simulink model "beam_control_ic_rx"  (R2022b)
settings: Solver=VariableStepAuto  StartTime=0.0  StopTime=136e-9  RelTol=1e-3
values from neighbouring files (symbols this model uses):
  Bias = 0    [ModelingRFSystemsWithAntennaArraysUsingAntennaBlockExample.m]    (also in beam_control_ic_rx_parameter.m)
  filter_gain0_0 = 0    [ModelingRFSystemsWithAntennaArraysUsingAntennaBlockExample.m]    (also in beam_control_ic_rx_parameter.m)
  filter_gain0_1 = 1/6    (= 0.166666666667)    [ModelingRFSystemsWithAntennaArraysUsingAntennaBlockExample.m]    (also in beam_control_ic_rx_parameter.m)
  filter_gain0_2 = 2/3    (= 0.666666666667)    [ModelingRFSystemsWithAntennaArraysUsingAntennaBlockExample.m]    (also in beam_control_ic_rx_parameter.m)
  filter_gain0_3 = 1/6    (= 0.166666666667)    [ModelingRFSystemsWithAntennaArraysUsingAntennaBlockExample.m]    (also in beam_control_ic_rx_parameter.m)
  filter_gain1_0 = 0    [ModelingRFSystemsWithAntennaArraysUsingAntennaBlockExample.m]    (also in beam_control_ic_rx_parameter.m)
  filter_gain1_1 = 1/2    (= 0.5)    [ModelingRFSystemsWithAntennaArraysUsingAntennaBlockExample.m]    (also in beam_control_ic_rx_parameter.m)
  filter_gain1_2 = 0    [ModelingRFSystemsWithAntennaArraysUsingAntennaBlockExample.m]    (also in beam_control_ic_rx_parameter.m)
  filter_gain1_3 = -1/2    (= -0.5)    [ModelingRFSystemsWithAntennaArraysUsingAntennaBlockExample.m]    (also in beam_control_ic_rx_parameter.m)
  filter_gain2_0 = 0    [ModelingRFSystemsWithAntennaArraysUsingAntennaBlockExample.m]    (also in beam_control_ic_rx_parameter.m)
  filter_gain2_1 = 1/2    (= 0.5)    [ModelingRFSystemsWithAntennaArraysUsingAntennaBlockExample.m]    (also in beam_control_ic_rx_parameter.m)
  filter_gain2_2 = -1    [ModelingRFSystemsWithAntennaArraysUsingAntennaBlockExample.m]    (also in beam_control_ic_rx_parameter.m)
  filter_gain2_3 = 1/2    (= 0.5)    [ModelingRFSystemsWithAntennaArraysUsingAntennaBlockExample.m]    (also in beam_control_ic_rx_parameter.m)
  filter_gain3_0 = 1/6    (= 0.166666666667)    [ModelingRFSystemsWithAntennaArraysUsingAntennaBlockExample.m]    (also in beam_control_ic_rx_parameter.m)
  filter_gain3_1 = -1/2    (= -0.5)    [ModelingRFSystemsWithAntennaArraysUsingAntennaBlockExample.m]    (also in beam_control_ic_rx_parameter.m)
  filter_gain3_2 = 1/2    (= 0.5)    [ModelingRFSystemsWithAntennaArraysUsingAntennaBlockExample.m]    (also in beam_control_ic_rx_parameter.m)
  filter_gain3_3 = -1/6    (= -0.166666666667)    [ModelingRFSystemsWithAntennaArraysUsingAntennaBlockExample.m]    (also in beam_control_ic_rx_parameter.m)
  fraction_delay = 1.5    [ModelingRFSystemsWithAntennaArraysUsingAntennaBlockExample.m]    (also in beam_control_ic_rx_parameter.m = 1)
  integer_delay = 0    [ModelingRFSystemsWithAntennaArraysUsingAntennaBlockExample.m]    (also in beam_control_ic_rx_parameter.m)
  N = 10    [ModelingRFSystemsWithAntennaArraysUsingAntennaBlockExample.m]    (also in beam_control_ic_rx_parameter.m)
  Ref = 2.048    [ModelingRFSystemsWithAntennaArraysUsingAntennaBlockExample.m]    (also in beam_control_ic_rx_parameter.m)
  rx_amplitude_compensation = 1    [ModelingRFSystemsWithAntennaArraysUsingAntennaBlockExample.m]    (also in beam_control_ic_rx_parameter.m)
  rx_freq_d_compensation = 250e6    (= 250000000)    [ModelingRFSystemsWithAntennaArraysUsingAntennaBlockExample.m]    (also in beam_control_ic_rx_parameter.m)
  rx_phase_compensation = 0    [ModelingRFSystemsWithAntennaArraysUsingAntennaBlockExample.m]    (also in beam_control_ic_rx_parameter.m)
undefined symbols (not defined in the file or in its folder): fdesignblkfcn, gcbh, pskmod
libraries: dspsigops x5, simulink_extras x3, dspmlti4 x3, msbDacArchitectures x2, commrfcorlib x1, commeq3 x1
(part 1 of 3)
settings Model: Creator=BOBO  LastModifiedBy=BOBO

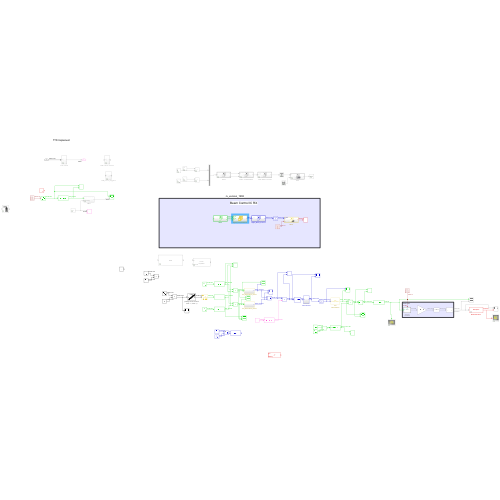
[thumbnail: Simulink's stored preview of the top-level diagram]
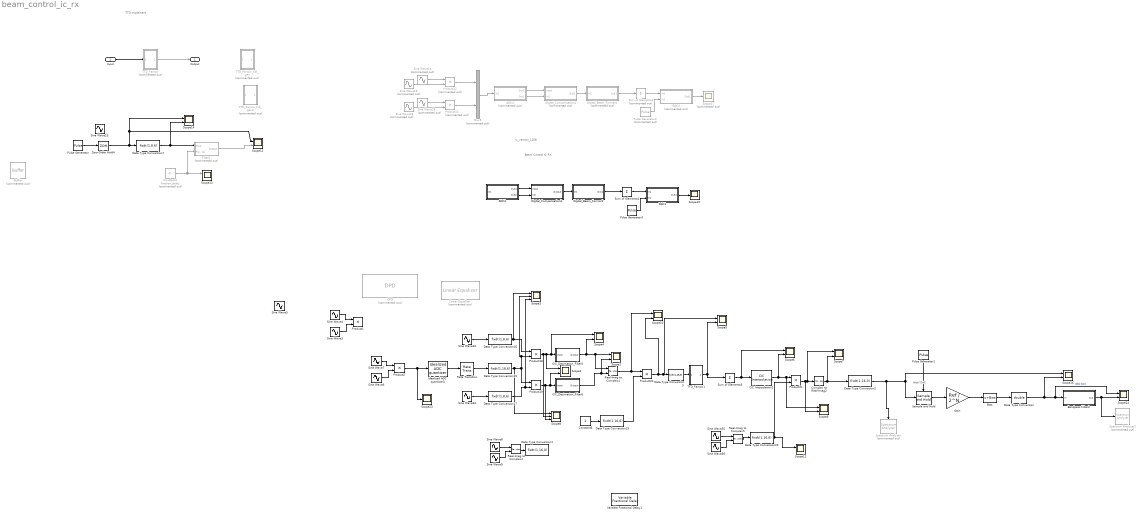
== system beam_control_ic_rx ==
  note: TTD Implement
  note: Ideal DAC
  note: rx_version_1208
  note: Beam Control IC RX
  Input : Inport
  ADC3 : Subsystem  TreatAsAtomicUnit=on
  ADC4 : Subsystem  Commented=on  TreatAsAtomicUnit=on
  Bandpass Filter3 : Subsystem  DialogController=fdesignblkfcn  InitFcn=fdesignblkfcn(gcbh, {'InitFcn'});  mask(Bandpass Filter){}
      mask help: Design a bandpass filter
      settings: CopyFcn=fdesignblkfcn(gcbh, {'CopyFcn'});
      mask Help: helpview(mapfilelocation('dsp'), 'dspbandpassfilter');
      mask Display: disp('Bandpass');
  Bias : Bias  Bias=Bias  SaturateOnIntegerOverflow=off
  Buffer : Buffer  Commented=on  OutputFrames=off
  CIC Interpolation2 : dspmlti4/CIC Interpolation  filtFrom=Dialog parameters  filtobj=Hm_interp  ftype=Interpolator  R=2  M=1  N=2  filterInternals=Full precision  BPS=[16 16 16 16]  FLPS=0  outputWordLength=32  outputFracLength=0  launchFVT=off  framing=Allow multirate processing  OutputFrames=off
      settings: LibrarySourceBlock=|
      | dsphdlsupportfiltering/CIC
      | Interpolation
  CIC_Decimation_Filter5 : Subsystem  Tag=FilterWizardSubSystem
      settings: ErrorFcn=dspFilterRealizedInBasicElemsAlgLoopErrFcnCallback
  CIC_Decimation_Filter6 : Subsystem  Tag=FilterWizardSubSystem
      settings: ErrorFcn=dspFilterRealizedInBasicElemsAlgLoopErrFcnCallback
  Complex to Real-Imag2 : ComplexToRealImag  Output=Real
  Constant4 : Constant  Commented=on  Value=fraction_delay  OutMin=0  OutMax=1  OutDataTypeStr=fixdt(1,16,10)
  Constant6 : Constant
  DAC3 : Subsystem  TreatAsAtomicUnit=on
  DAC4 : Subsystem  Commented=on  TreatAsAtomicUnit=on
  DPD : commrfcorlib/DPD  Commented=on  PolynomialType=Memory polynomial  CoefficientSource=Property  Coefficients=complex([1 0 0 0 0; 0 0 0 0 0; 0 0 0 0 0])  SimulateUsing=Code generation
  Data Type Conversion : DataTypeConversion  OutDataTypeStr=double  SaturateOnIntegerOverflow=off  RndMeth=Floor
  Data Type Conversion1 : DataTypeConversion  OutDataTypeStr=fixdt(1,16,0)  SaturateOnIntegerOverflow=off  RndMeth=Floor
  Data Type Conversion{3,15,19..20} (4 alike) : DataTypeConversion  OutDataTypeStr=fixdt(1,16,6)  SaturateOnIntegerOverflow=off  RndMeth=Floor
  Data Type Conversion16 : DataTypeConversion  OutDataTypeStr=fixdt(1,8,6)  SaturateOnIntegerOverflow=off  RndMeth=Floor
  Data Type Conversion17 : DataTypeConversion  OutDataTypeStr=fixdt(1,8,6)  SaturateOnIntegerOverflow=off  RndMeth=Floor
  Data Type Conversion2 : DataTypeConversion  OutDataTypeStr=fixdt(1,16,0)  SaturateOnIntegerOverflow=off  RndMeth=Floor
  Data Type Conversion7 : DataTypeConversion  OutMin=-1  OutMax=0.99  OutDataTypeStr=fixdt(1,8,6)  SaturateOnIntegerOverflow=off  RndMeth=Floor
  Digital_Beam_Former3 : Subsystem  TreatAsAtomicUnit=on
  Digital_Beam_Former4 : Subsystem  Commented=on  TreatAsAtomicUnit=on
  Digital_Compensation3 : Subsystem  TreatAsAtomicUnit=on
  Digital_Compensation4 : Subsystem  Commented=on  TreatAsAtomicUnit=on
  Filter1 : Subsystem  Tag=FilterWizardSubSystem  Commented=on
      settings: ErrorFcn=dspFilterRealizedInBasicElemsAlgLoopErrFcnCallback
  Gain : Gain  Gain=Ref / 2^N
  Idealized ADC quantizer3 : simulink_extras/Additional Discrete/Idealized ADC quantizer  NumberOfConverterBits=8  Vmin=-1  Vmax=1  OutputDataType=double  OutputNegativeValues=on
  Linear Equalizer : commeq3/Linear Equalizer  Commented=on  NumTaps=5  Constellation=pskmod( 0:3, 4, pi/4, 'bin' )  InputSamplesPerSymbol=1  Algorithm=LMS  StepSize=0.01  ForgettingFactor=0.99  InitialInverseCorrelationMatrix=0.1  ReferenceTap=3  InputDelay=0  AdaptWeightsSource=Property  AdaptWeights=on  InitialWeightsSource=Auto  InitialWeights=0  TrainingInitialWeights=0  BlindInitialWeights=[ 0; 0; 1; 0; 0 ]  WeightUpdatePeriod=1  TrainingFlagInputPort=off  AdaptAfterTraining=on  ResetInputPort=off  ErrorOutputPort=off  TapWeightsOutputPort=off  SimulateUsing=Code generation
  Mux5 : Mux  Commented=on  Inputs=2
  Product{1..2,18..21} (6 alike) : Product
  Product11 : Product  Commented=on
  Product12 : Product  Commented=on
  Pulse Generator : DiscretePulseGenerator  PulseType=Time based  Period=5e-9  PulseWidth=50
  Pulse Generator1 : DiscretePulseGenerator  PulseType=Time based  Period=1/1e9  PulseWidth=50
  Pulse Generator2 : DiscretePulseGenerator  Commented=on  PulseType=Time based  Period=1/1e9  PulseWidth=50
  Pulse Generator3 : DiscretePulseGenerator  PulseType=Time based  Period=1/1e9  PulseWidth=50
  Rate Transition : RateTransition  OutPortSampleTime=1/1e9
  Real-Imag to Complex2 : RealImagToComplex
  Real-Imag to Complex4 : RealImagToComplex
  Real-Imag to Complex5 : RealImagToComplex
  Sample and Hold : dspsigops/Sample and Hold  trig=Rising edge  initCond=0  latchinput=off
  Scope{1..2,4..7,9..14,16,24} (14 alike) : Scope  NumInputPorts=2
  Scope15 : Scope
  Scope17 : Scope  Commented=on
  Scope23 : Scope
  Scope3 : Scope  NumInputPorts=3
  Scope8 : Scope  NumInputPorts=3
  Sine Wave14 : Sin  Commented=on  Frequency=2*pi*3.25e9  SampleTime=0
  Sine Wave19 : Sin  Commented=on  Frequency=2*pi*62.5e6  SampleTime=0
  Sine Wave23 : Sin  Frequency=2*pi*3.25e9  SampleTime=1e-11
  Sine Wave24 : Sin  Commented=on  Frequency=2*pi*3.25e9  SampleTime=0
  Sine Wave26 : Sin  Commented=on  Frequency=2*pi*62.5e6  SampleTime=0
  Sine Wave3 : Sin  Frequency=2*pi*62.5e6  SampleTime=0
  Sine Wave33 : Sin  Frequency=2*pi*250e6  Phase=1.57  SampleTime=1/1e9
  Sine Wave34 : Sin  Frequency=2*pi*250e6  SampleTime=1/1e9
  Sine Wave35 : Sin  Frequency=2*pi*250e6  Phase=1.57  SampleTime=1/1e9
  Sine Wave36 : Sin  Frequency=2*pi*250e6  SampleTime=1/1e9
  Sine Wave4 : Sin  Frequency=2*pi*3.25e9  SampleTime=0
  Sine Wave5 : Sin  Frequency=2*pi*3.25e9  SampleTime=0
  Sine Wave6 : Sin  Frequency=2*pi*62.5e6  SampleTime=0
  Sine Wave7 : Sin  Frequency=2*pi*3.25e9  SampleTime=0
  Sine Wave8 : Sin  Amplitude=rx_amplitude_compensation  Frequency=2*pi*rx_freq_d_compensation  Phase=pi*(rx_phase_compensation+90)/180  SampleTime=1/5e8
  Sine Wave9 : Sin  Amplitude=rx_amplitude_compensation  Frequency=2*pi*rx_freq_d_compensation  Phase=pi*rx_phase_compensation/180  SampleTime=1/5e8
  Spectrum Analyzer : SpectrumAnalyzer  Commented=on
  Spectrum Analyzer2 : SpectrumAnalyzer  Commented=on
  Sum of Elements1 : Sum  Inputs=+
  Sum of Elements4 : Sum  Commented=on  Inputs=+
  Sum of Elements5 : Sum  Inputs=+
  TTD_Farrow : Subsystem  Commented=on
  TTD_Farrow1 : Subsystem
  TTD_Farrow_hdl_gen : Subsystem  Commented=on
  TTD_Farrow_hdl_gen2 : Subsystem  Commented=on
  Variable Fractional Delay1 : dspsigops/Variable Fractional Delay  mode=OBSOLETE  modeActive=Linear  L=4  FarrowL=4  R=10  alpha=1  dmax=100  InputProcessing=Columns as channels (frame based)  ic=0  noDFT=off  fallbackFIR=Clip to the minimum value necessary for centered kernel  fallbackFarrow=Clip to the minimum value necessary for centered kernel  roundingMode=Zero  overflowMode=off
  Zero-Order Hold4 : ZeroOrderHold  SampleTime=1e-9
  Output : Outport
  wires:
  Input/1 -> TTD_Farrow/1(In1)
  TTD_Farrow/1(Output) -> Output/1
  Pulse Generator/1 -> Zero-Order Hold4/1
  Data Type Conversion7/1 -> Filter1/1(Input), Scope14/2
  Filter1/1(Output) -> Scope12/2
  Zero-Order Hold4/1 -> Scope14/1, Scope12/1, Data Type Conversion7/1
  Constant4/1 -> Filter1/2(FracDelay), Scope13/1
  Idealized ADC quantizer3/1 -> Rate Transition/1
  Rate Transition/1 -> Data Type Conversion15/1
  Sine Wave33/1 -> Data Type Conversion16/1
  Sine Wave34/1 -> Data Type Conversion17/1
  Data Type Conversion16/1 -> Product18/1, Scope3/1
  Data Type Conversion15/1 -> Scope8/1, Product19/1, Product18/2, Scope3/2
  Data Type Conversion17/1 -> Scope3/3, Product19/2
  Product18/1 -> Scope2/1, Scope4/1, CIC_Decimation_Filter5/1(Input), Scope8/2
  Product19/1 -> Scope8/3, Scope2/2, CIC_Decimation_Filter6/1(Input)
  CIC_Decimation_Filter5/1(Output) -> Scope4/2, Real-Imag to Complex4/1, Scope1/1
  CIC_Decimation_Filter6/1(Output) -> Scope1/2, Real-Imag to Complex4/2
  Real-Imag to Complex4/1 -> Scope10/1, Product20/1
  Data Type Conversion19/1 -> Product20/2
  Constant6/1 -> Data Type Conversion19/1
  Product20/1 -> Scope10/2, Scope5/1, Data Type Conversion3/1
  Sum of Elements5/1 -> Scope6/1, CIC Interpolation2/1
  CIC Interpolation2/1 -> Scope6/2, Scope9/1, Product21/1
  Sine Wave35/1 -> Real-Imag to Complex5/1
  Real-Imag to Complex5/1 -> Data Type Conversion20/1
  Sine Wave36/1 -> Real-Imag to Complex5/2
  Product21/1 -> Scope9/2, Scope7/1, Complex to Real-Imag2/1
  Complex to Real-Imag2/1 -> Scope7/2, Data Type Conversion2/1
  Pulse Generator1/1 -> Sample and Hold/Trigger
  Gain/1 -> Bias/1
  Bias/1 -> Data Type Conversion/1
  Sample and Hold/1 -> Gain/1
  Data Type Conversion2/1 -> Scope16/1, Sample and Hold/1, Spectrum Analyzer/1
  Data Type Conversion/1 -> Scope16/2, Scope24/1, Bandpass Filter3/1(In)  "Ideal DAC"
  Product12/1 -> Mux5/1
  Sine Wave14/1 -> Product12/1
  Sine Wave19/1 -> Product12/2
  Sine Wave26/1 -> Product11/2
  Sine Wave24/1 -> Product11/1
  Product11/1 -> Mux5/2
  Mux5/1 -> ADC4/1(In1)
  Digital_Compensation4/1(Out1) -> Digital_Beam_Former4/1(In1)
  ADC4/2(Out2) -> Digital_Compensation4/2(In2)
  ADC4/1(Out1) -> Digital_Compensation4/1(Input)
  DAC4/1(Out1) -> Scope17/1
  Sum of Elements4/1 -> DAC4/1(In1)
  Digital_Beam_Former4/1(Out1) -> Sum of Elements4/1
  Bandpass Filter3/1(Out) -> Spectrum Analyzer2/1, Scope24/2
  Pulse Generator2/1 -> DAC4/2(In2)
  Sine Wave3/1 -> Product1/2
  Sine Wave4/1 -> Product1/1
  Digital_Beam_Former3/1(Out1) -> Sum of Elements1/1
  Pulse Generator3/1 -> DAC3/2(In2)
  DAC3/1(Out1) -> Scope15/1
  Digital_Compensation3/1(Output) -> Digital_Beam_Former3/1(In1)
  Sum of Elements1/1 -> DAC3/1(In1)
  ADC3/2(Out2) -> Digital_Compensation3/2(In2)
  ADC3/1(Out1) -> Digital_Compensation3/1(Input)
  Data Type Conversion20/1 -> Product21/2, Scope11/1
  Sine Wave7/1 -> Product2/1
  Sine Wave6/1 -> Product2/2
  Product2/1 -> Scope23/1, Idealized ADC quantizer3/1
  Sine Wave8/1 -> Real-Imag to Complex2/1
  Sine Wave9/1 -> Real-Imag to Complex2/2
  Real-Imag to Complex2/1 -> Data Type Conversion1/1
  Data Type Conversion3/1 -> TTD_Farrow1/1(In1)
  TTD_Farrow1/1(Output) -> Sum of Elements5/1, Scope5/2

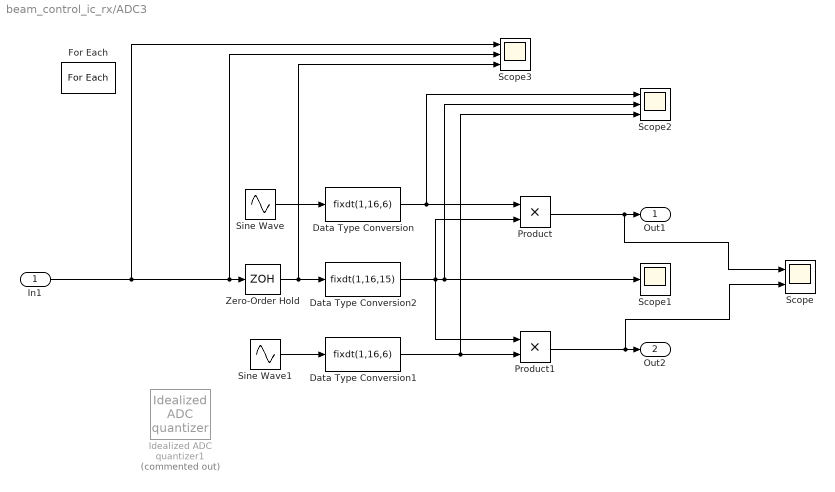
== system beam_control_ic_rx/ADC3 ==
  In1 : Inport  Partition=on  PartitionDimension=1  PartitionWidth=1  PartitionOffset=0
  Data Type Conversion : DataTypeConversion  OutMin=-1  OutMax=1  OutDataTypeStr=fixdt(1,16,6)  SaturateOnIntegerOverflow=off  RndMeth=Floor
  Data Type Conversion1 : DataTypeConversion  OutMin=-1  OutMax=1  OutDataTypeStr=fixdt(1,16,6)  SaturateOnIntegerOverflow=off  RndMeth=Floor
  Data Type Conversion2 : DataTypeConversion  OutMin=-1  OutMax=0.9  OutDataTypeStr=fixdt(1,16,15)  SaturateOnIntegerOverflow=off  RndMeth=Floor
  For Each : ForEach  DisableCoverage=on
  Idealized ADC quantizer1 : simulink_extras/Additional Discrete/Idealized ADC quantizer  Commented=on  NumberOfConverterBits=12  Vmin=-5  Vmax=5  OutputDataType=double  OutputNegativeValues=on
  Product : Product
  Product1 : Product
  Scope : Scope  NumInputPorts=2
  Scope1 : Scope
  Scope2 : Scope  NumInputPorts=3
  Scope3 : Scope  NumInputPorts=3
  Sine Wave : Sin  Frequency=2*pi*250e6  Phase=1.57  SampleTime=1/1e9
  Sine Wave1 : Sin  Frequency=2*pi*250e6  SampleTime=1/1e9
  Zero-Order Hold : ZeroOrderHold  SampleTime=1/1e9
  Out1 : Outport  ConcatenationDimension=1
  Out2 : Outport  Port=2  ConcatenationDimension=1
  wires:
  Data Type Conversion1/1 -> Scope2/3, Product1/2
  In1/1 -> Scope3/2, Zero-Order Hold/1, Scope3/1
  Sine Wave/1 -> Data Type Conversion/1
  Sine Wave1/1 -> Data Type Conversion1/1
  Zero-Order Hold/1 -> Scope3/3, Data Type Conversion2/1
  Data Type Conversion/1 -> Product/1, Scope2/1
  Data Type Conversion2/1 -> Scope1/1, Scope2/2, Product1/1, Product/2
  Product/1 -> Scope/1, Out1/1
  Product1/1 -> Scope/2, Out2/1

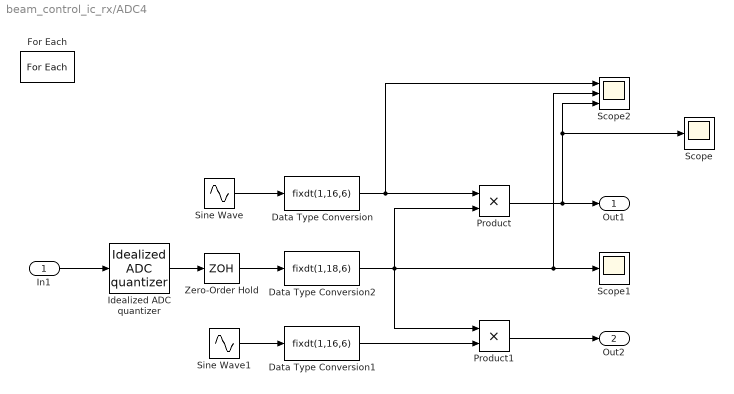
== system beam_control_ic_rx/ADC4 ==
  In1 : Inport  Partition=on  PartitionDimension=1  PartitionWidth=1  PartitionOffset=0
  Data Type Conversion : DataTypeConversion  OutMin=-1  OutMax=1  OutDataTypeStr=fixdt(1,16,6)  SaturateOnIntegerOverflow=off  RndMeth=Floor
  Data Type Conversion1 : DataTypeConversion  OutMin=-1  OutMax=1  OutDataTypeStr=fixdt(1,16,6)  SaturateOnIntegerOverflow=off  RndMeth=Floor
  Data Type Conversion2 : DataTypeConversion  OutMin=-2048  OutMax=2047  OutDataTypeStr=fixdt(1,18,6)  SaturateOnIntegerOverflow=off  RndMeth=Floor
  For Each : ForEach  DisableCoverage=on
  Idealized ADC quantizer : simulink_extras/Additional Discrete/Idealized ADC quantizer  NumberOfConverterBits=12  Vmin=-1  Vmax=1  OutputDataType=double  OutputNegativeValues=on
  Product : Product
  Product1 : Product
  Scope : Scope
  Scope1 : Scope
  Scope2 : Scope  NumInputPorts=3
  Sine Wave : Sin  Frequency=2*pi*250e6  Phase=1.57  SampleTime=1/1e9
  Sine Wave1 : Sin  Frequency=2*pi*250e6  SampleTime=1/1e9
  Zero-Order Hold : ZeroOrderHold  SampleTime=1/1e9
  Out1 : Outport  ConcatenationDimension=1
  Out2 : Outport  Port=2  ConcatenationDimension=1
  wires:
  Product1/1 -> Out2/1
  Product/1 -> Scope/1, Scope2/3, Out1/1
  Data Type Conversion2/1 -> Product/2, Product1/1, Scope2/2, Scope1/1
  Data Type Conversion/1 -> Scope2/1, Product/1
  Zero-Order Hold/1 -> Data Type Conversion2/1
  Sine Wave1/1 -> Data Type Conversion1/1
  Sine Wave/1 -> Data Type Conversion/1
  Idealized ADC quantizer/1 -> Zero-Order Hold/1
  In1/1 -> Idealized ADC quantizer/1
  Data Type Conversion1/1 -> Product1/2

== system beam_control_ic_rx/Bandpass Filter3 ==
  In : Inport
  Generated Filter Block : DiscreteFir  Tag=BlockMethodSubSystem  Coefficients=[-0.000551445390270867506 0.000407430436883946413 0.00151170095910276784 0.00170809108636746755 -0.000183233989486140172 -0.00314427517439309695 -0.00408384949539862194 -0.000859536641631024833 0.00458828280495307203 0.00703118910578414639 0.00304274168675388234 -0.00462111674625677576 -0.00882607470501511893 -0.00522014043057489156 0.00277191525149639382 0.00730259808984131537 0.00474853789832731764 -0.000332137279825720844 -0.00125943108082663064 0.001596135152078317 0.000647809790796010439 -0.00801520700503077603 -0.0156681967330769729 -0.00792830354994228381 0.0163284487042885569 0.0360058824865698776 0.0248375883164067765 -0.0180029551213413963 -0.0572925026311378038 -0.0501414407980040541 0.00875479098791274307 0.0720308491137559154 0.0780256286801277177 0.0114831560658058014 -0.0739106277220435842 -0.0999313296142419205 -0.0376048498748084298 0.0611143159293767238 0.108245533083798362 0.0611143159293767238 -0.0376048498748084298 -0.0999313296142419205 -0.0739106277220435842 0.0114831560658058014 0.0780256286801277177 0.0720308491137559154 0.00875479098791274307 -0.0501414407980040541 -0.0572925026311378038 -0.0180029551213413963 0.0248375883164067765 0.0360058824865698776 0.0163284487042885569 -0.00792830354994228381 -0.0156681967330769729 -0.00801520700503077603 0.000647809790796010439 0.001596135152078317 -0.00125943108082663064 -0.000332137279825720844 0.00474853789832731764 0.00730259808984131537 0.00277191525149639382 -0.00522014043057489156 -0.00882607470501511893 -0.00462111674625677576 0.00304274168675388234 0.00703118910578414639 0.00458828280495307203 -0.000859536641631024833 -0.00408384949539862194 -0.00314427517439309695 -0.000183233989486140172 0.00170809108636746755 0.00151170095910276784 0.000407430436883946413 -0.000551445390270867506]  InputProcessing=Columns as channels (frame based)
  Out : Outport  VectorParamsAs1DForOutWhenUnconnected=off
  wires:
  Generated Filter Block/1 -> Out/1
  In/1 -> Generated Filter Block/1

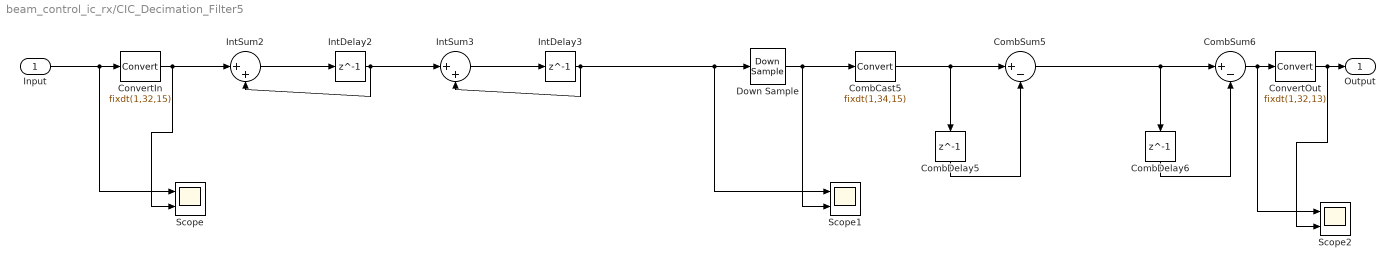
== system beam_control_ic_rx/CIC_Decimation_Filter5 ==
  Input : Inport
  CombCast5 : DataTypeConversion  OutDataTypeStr=fixdt(1,34,15)  SaturateOnIntegerOverflow=off  RndMeth=Floor
  CombDelay5 : Delay  DelayLength=1  InitialCondition=0
  CombDelay6 : Delay  DelayLength=1  InitialCondition=0
  CombSum5 : Sum  Inputs=|+-  AccumDataTypeStr=fixdt(1,34,15)  OutDataTypeStr=fixdt(1,34,15)
  CombSum6 : Sum  Inputs=|+-  AccumDataTypeStr=fixdt(1,34,15)  OutDataTypeStr=fixdt(1,34,15)
  ConvertIn : DataTypeConversion  OutDataTypeStr=fixdt(1,32,15)  RndMeth=Nearest
  ConvertOut : DataTypeConversion  OutDataTypeStr=fixdt(1,32,13)  SaturateOnIntegerOverflow=off  RndMeth=Floor
  Down Sample : DownSample  RateOptions=Allow multirate processing  AllowArbitraryFixedInput=on
  IntDelay2 : Delay  DelayLength=1  InitialCondition=0
  IntDelay3 : Delay  DelayLength=1  InitialCondition=0
  IntSum2 : Sum  Inputs=|++  AccumDataTypeStr=fixdt(1,34,15)  OutDataTypeStr=fixdt(1,34,15)
  IntSum3 : Sum  Inputs=|++  AccumDataTypeStr=fixdt(1,34,15)  OutDataTypeStr=fixdt(1,34,15)
  Scope : Scope  NumInputPorts=2
  Scope1 : Scope  NumInputPorts=2
  Scope2 : Scope  NumInputPorts=2
  Output : Outport
  wires:
  Input/1 -> Scope/1, ConvertIn/1
  ConvertIn/1 -> Scope/2, IntSum2/1
  IntSum2/1 -> IntDelay2/1
  IntDelay2/1 -> IntSum2/2, IntSum3/1
  IntSum3/1 -> IntDelay3/1
  IntDelay3/1 -> IntSum3/2, Scope1/1, Down Sample/1
  Down Sample/1 -> Scope1/2, CombCast5/1
  CombSum5/1 -> CombSum6/1, CombDelay6/1
  CombDelay5/1 -> CombSum5/2
  CombCast5/1 -> CombSum5/1, CombDelay5/1
  CombSum6/1 -> Scope2/1, ConvertOut/1
  CombDelay6/1 -> CombSum6/2
  ConvertOut/1 -> Scope2/2, Output/1

== system beam_control_ic_rx/CIC_Decimation_Filter6 ==
  Input : Inport
  CombCast5 : DataTypeConversion  OutDataTypeStr=fixdt(1,34,15)  SaturateOnIntegerOverflow=off  RndMeth=Floor
  CombDelay5 : Delay  DelayLength=1  InitialCondition=0
  CombDelay6 : Delay  DelayLength=1  InitialCondition=0
  CombSum5 : Sum  Inputs=|+-  AccumDataTypeStr=fixdt(1,34,15)  OutDataTypeStr=fixdt(1,34,15)
  CombSum6 : Sum  Inputs=|+-  AccumDataTypeStr=fixdt(1,34,15)  OutDataTypeStr=fixdt(1,34,15)
  ConvertIn : DataTypeConversion  OutDataTypeStr=fixdt(1,32,15)  RndMeth=Nearest
  ConvertOut : DataTypeConversion  OutDataTypeStr=fixdt(1,32,13)  SaturateOnIntegerOverflow=off  RndMeth=Floor
  Down Sample : DownSample  RateOptions=Allow multirate processing  AllowArbitraryFixedInput=on
  IntDelay2 : Delay  DelayLength=1  InitialCondition=0
  IntDelay3 : Delay  DelayLength=1  InitialCondition=0
  IntSum2 : Sum  Inputs=|++  AccumDataTypeStr=fixdt(1,34,15)  OutDataTypeStr=fixdt(1,34,15)
  IntSum3 : Sum  Inputs=|++  AccumDataTypeStr=fixdt(1,34,15)  OutDataTypeStr=fixdt(1,34,15)
  Output : Outport
  wires:
  ConvertOut/1 -> Output/1
  CombDelay6/1 -> CombSum6/2
  CombSum6/1 -> ConvertOut/1
  CombCast5/1 -> CombDelay5/1, CombSum5/1
  CombDelay5/1 -> CombSum5/2
  CombSum5/1 -> CombDelay6/1, CombSum6/1
  Down Sample/1 -> CombCast5/1
  IntDelay3/1 -> Down Sample/1, IntSum3/2
  IntSum3/1 -> IntDelay3/1
  IntDelay2/1 -> IntSum3/1, IntSum2/2
  IntSum2/1 -> IntDelay2/1
  ConvertIn/1 -> IntSum2/1
  Input/1 -> ConvertIn/1

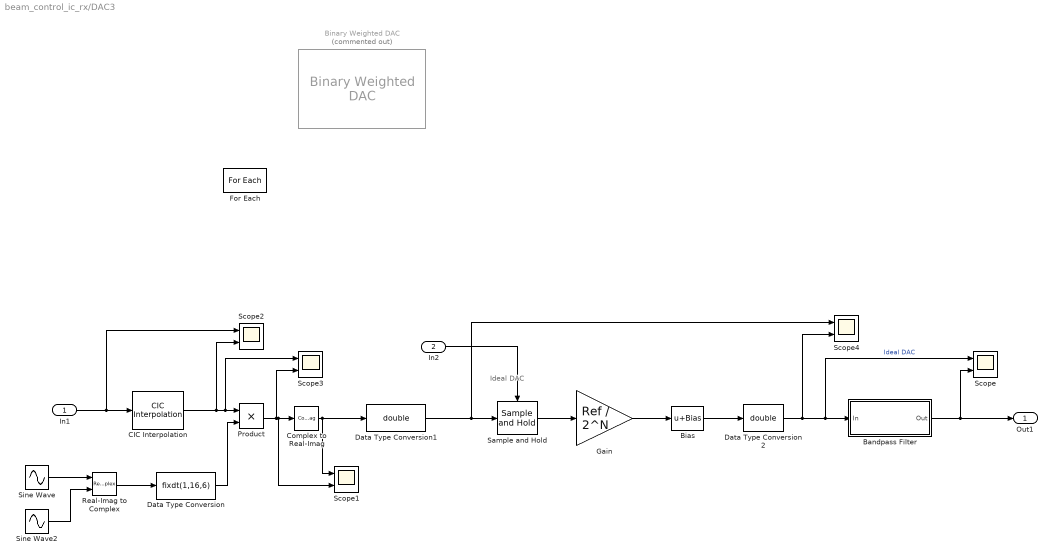
== system beam_control_ic_rx/DAC3 ==
  note: Ideal DAC
  In1 : Inport  Partition=on  PartitionDimension=1  PartitionWidth=1  PartitionOffset=0
  In2 : Inport  Port=2  Partition=on  PartitionDimension=1  PartitionWidth=1  PartitionOffset=0
  Bandpass Filter : Subsystem  DialogController=fdesignblkfcn  InitFcn=fdesignblkfcn(gcbh, {'InitFcn'});  mask(Bandpass Filter){}
      mask help: Design a bandpass filter
      settings: CopyFcn=fdesignblkfcn(gcbh, {'CopyFcn'});
      mask Help: helpview(mapfilelocation('dsp'), 'dspbandpassfilter');
      mask Display: disp('Bandpass');
  Bias : Bias  Bias=Bias  SaturateOnIntegerOverflow=off
  Binary Weighted DAC : msbDacArchitectures/Binary Weighted DAC  Commented=on  NBits=5  Polarity=Bipolar  ExtStartClk=on  StartFreq=1e6  Ref=2  Bias=0  ReadySignal=off  EnableLinearityImpairments=on  OffsetError=0  OffsetErrorUnit=LSB  GainError=0  GainErrorUnit=LSB  EnableTimingImpairments=on  TimingSpecification=Settling time  SettlingTime=2e-7  SettlingTimeTolerance=0.5  RisingSlewRate=5015625  FallingSlewRate=-5015625
  CIC Interpolation : dspmlti4/CIC Interpolation  filtFrom=Dialog parameters  filtobj=Hm_interp  ftype=Interpolator  R=2  M=1  N=2  filterInternals=Full precision  BPS=[16 16 16 16]  FLPS=0  outputWordLength=32  outputFracLength=0  launchFVT=off  framing=Allow multirate processing  OutputFrames=off
      settings: LibrarySourceBlock=|
      | dsphdlsupportfiltering/CIC
      | Interpolation
  Complex to Real-Imag : ComplexToRealImag  Output=Real
  Data Type Conversion : DataTypeConversion  OutDataTypeStr=fixdt(1,16,6)  SaturateOnIntegerOverflow=off  RndMeth=Floor
  Data Type Conversion1 : DataTypeConversion  OutDataTypeStr=double  SaturateOnIntegerOverflow=off  RndMeth=Floor
  Data Type Conversion2 : DataTypeConversion  OutDataTypeStr=double  SaturateOnIntegerOverflow=off  RndMeth=Floor
  For Each : ForEach  DisableCoverage=on
  Gain : Gain  Gain=Ref / 2^N
  Product : Product
  Real-Imag to Complex : RealImagToComplex
  Sample and Hold : dspsigops/Sample and Hold  trig=Rising edge  initCond=0  latchinput=off
  Scope{,1..4} (5 alike) : Scope  NumInputPorts=2
  Sine Wave : Sin  Frequency=2*pi*250e6  Phase=1.57  SampleTime=1/1e9
  Sine Wave2 : Sin  Frequency=2*pi*250e6  SampleTime=1/1e9
  Out1 : Outport  ConcatenationDimension=1
  wires:
  Bandpass Filter/1(Out) -> Out1/1, Scope/2
  In2/1 -> Sample and Hold/Trigger
  Sample and Hold/1 -> Gain/1
  Gain/1 -> Bias/1
  Bias/1 -> Data Type Conversion2/1
  Data Type Conversion1/1 -> Sample and Hold/1, Scope4/1
  Data Type Conversion2/1 -> Bandpass Filter/1(In), Scope/1, Scope4/2  "Ideal DAC"
  Real-Imag to Complex/1 -> Data Type Conversion/1
  Sine Wave2/1 -> Real-Imag to Complex/2
  Sine Wave/1 -> Real-Imag to Complex/1
  In1/1 -> CIC Interpolation/1, Scope2/1
  CIC Interpolation/1 -> Scope3/1, Product/1, Scope2/2
  Product/1 -> Scope3/2, Complex to Real-Imag/1, Scope1/2
  Complex to Real-Imag/1 -> Scope1/1, Data Type Conversion1/1
  Data Type Conversion/1 -> Product/2

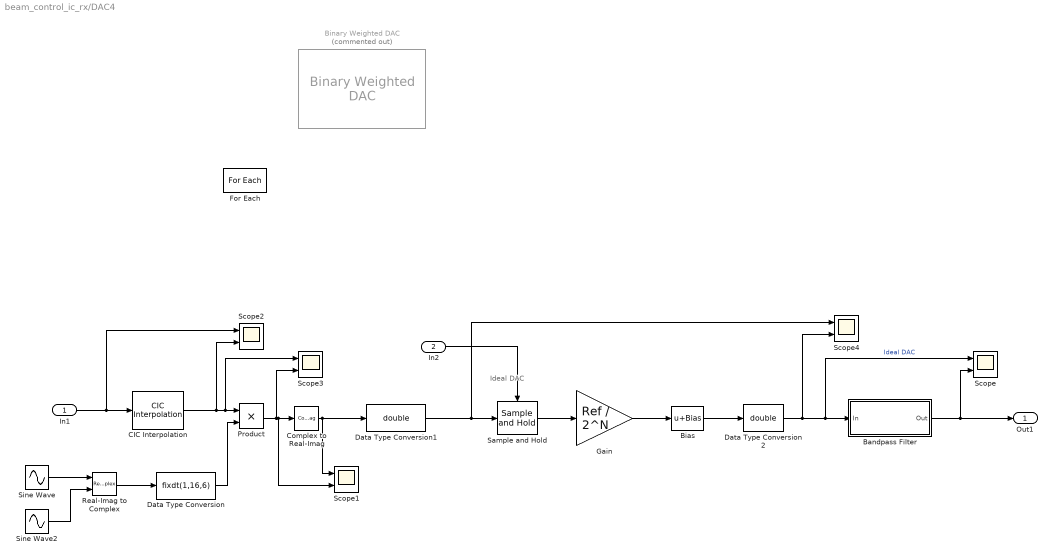
== system beam_control_ic_rx/DAC4 ==
  note: Ideal DAC
  In1 : Inport  Partition=on  PartitionDimension=1  PartitionWidth=1  PartitionOffset=0
  In2 : Inport  Port=2  Partition=on  PartitionDimension=1  PartitionWidth=1  PartitionOffset=0
  Bandpass Filter : Subsystem  DialogController=fdesignblkfcn  InitFcn=fdesignblkfcn(gcbh, {'InitFcn'});  mask(Bandpass Filter){}
      mask help: Design a bandpass filter
      settings: CopyFcn=fdesignblkfcn(gcbh, {'CopyFcn'});
      mask Help: helpview(mapfilelocation('dsp'), 'dspbandpassfilter');
      mask Display: disp('Bandpass');
  Bias : Bias  Bias=Bias  SaturateOnIntegerOverflow=off
  Binary Weighted DAC : msbDacArchitectures/Binary Weighted DAC  Commented=on  NBits=5  Polarity=Bipolar  ExtStartClk=on  StartFreq=1e6  Ref=2  Bias=0  ReadySignal=off  EnableLinearityImpairments=on  OffsetError=0  OffsetErrorUnit=LSB  GainError=0  GainErrorUnit=LSB  EnableTimingImpairments=on  TimingSpecification=Settling time  SettlingTime=2e-7  SettlingTimeTolerance=0.5  RisingSlewRate=5015625  FallingSlewRate=-5015625
  CIC Interpolation : dspmlti4/CIC Interpolation  filtFrom=Dialog parameters  filtobj=Hm_interp  ftype=Interpolator  R=2  M=1  N=2  filterInternals=Full precision  BPS=[16 16 16 16]  FLPS=0  outputWordLength=32  outputFracLength=0  launchFVT=off  framing=Allow multirate processing  OutputFrames=off
      settings: LibrarySourceBlock=|
      | dsphdlsupportfiltering/CIC
      | Interpolation
  Complex to Real-Imag : ComplexToRealImag  Output=Real
  Data Type Conversion : DataTypeConversion  OutDataTypeStr=fixdt(1,16,6)  SaturateOnIntegerOverflow=off  RndMeth=Floor
  Data Type Conversion1 : DataTypeConversion  OutDataTypeStr=double  SaturateOnIntegerOverflow=off  RndMeth=Floor
  Data Type Conversion2 : DataTypeConversion  OutDataTypeStr=double  SaturateOnIntegerOverflow=off  RndMeth=Floor
  For Each : ForEach  DisableCoverage=on
  Gain : Gain  Gain=Ref / 2^N
  Product : Product
  Real-Imag to Complex : RealImagToComplex
  Sample and Hold : dspsigops/Sample and Hold  trig=Rising edge  initCond=0  latchinput=off
  Scope{,1..4} (5 alike) : Scope  NumInputPorts=2
  Sine Wave : Sin  Frequency=2*pi*250e6  Phase=1.57  SampleTime=1/1e9
  Sine Wave2 : Sin  Frequency=2*pi*250e6  SampleTime=1/1e9
  Out1 : Outport  ConcatenationDimension=1
  wires:
  Data Type Conversion/1 -> Product/2
  Complex to Real-Imag/1 -> Data Type Conversion1/1, Scope1/1
  Product/1 -> Scope1/2, Complex to Real-Imag/1, Scope3/2
  CIC Interpolation/1 -> Scope2/2, Product/1, Scope3/1
  In1/1 -> Scope2/1, CIC Interpolation/1
  Sine Wave/1 -> Real-Imag to Complex/1
  Sine Wave2/1 -> Real-Imag to Complex/2
  Real-Imag to Complex/1 -> Data Type Conversion/1
  Data Type Conversion2/1 -> Scope4/2, Scope/1, Bandpass Filter/1(In)  "Ideal DAC"
  Data Type Conversion1/1 -> Scope4/1, Sample and Hold/1
  Bias/1 -> Data Type Conversion2/1
  Gain/1 -> Bias/1
  Sample and Hold/1 -> Gain/1
  In2/1 -> Sample and Hold/Trigger
  Bandpass Filter/1(Out) -> Scope/2, Out1/1

== system beam_control_ic_rx/Digital_Beam_Former3 ==
  In1 : Inport  Partition=on  PartitionDimension=1  PartitionWidth=1  PartitionOffset=0
  For Each : ForEach  DisableCoverage=on
  Gain : Gain  OutDataTypeStr=Inherit: Same as input
  Out1 : Outport  ConcatenationDimension=1
  wires:
  In1/1 -> Gain/1
  Gain/1 -> Out1/1

== system beam_control_ic_rx/Digital_Beam_Former4 ==
  In1 : Inport  Partition=on  PartitionDimension=1  PartitionWidth=1  PartitionOffset=0
  For Each : ForEach  DisableCoverage=on
  Gain : Gain  OutDataTypeStr=Inherit: Same as input
  Out1 : Outport  ConcatenationDimension=1
  wires:
  Gain/1 -> Out1/1
  In1/1 -> Gain/1

== system beam_control_ic_rx/Digital_Compensation3 ==
  Input : Inport  Partition=on  PartitionDimension=1  PartitionWidth=1  PartitionOffset=0
  In2 : Inport  Port=2  Partition=on  PartitionDimension=1  PartitionWidth=1  PartitionOffset=0
  CIC_Decimation_Filter1 : Subsystem  Tag=FilterWizardSubSystem
      settings: ErrorFcn=dspFilterRealizedInBasicElemsAlgLoopErrFcnCallback
  CIC_Decimation_Filter2 : Subsystem  Tag=FilterWizardSubSystem
      settings: ErrorFcn=dspFilterRealizedInBasicElemsAlgLoopErrFcnCallback
  Constant : Constant
  Data Type Conversion : DataTypeConversion  OutDataTypeStr=fixdt(1,16,0)  SaturateOnIntegerOverflow=off  RndMeth=Floor
  Data Type Conversion3 : DataTypeConversion  OutDataTypeStr=fixdt(1,16,6)  SaturateOnIntegerOverflow=off  RndMeth=Floor
  For Each : ForEach  DisableCoverage=on
  Product : Product
  Real-Imag to Complex : RealImagToComplex
  Scope : Scope  NumInputPorts=2
  Scope1 : Scope  NumInputPorts=2
  Scope2 : Scope  NumInputPorts=2
  Scope3 : Scope  NumInputPorts=3
  TTD_Farrow1 : Subsystem
  Output : Outport  ConcatenationDimension=1
  wires:
  Input/1 -> Scope2/1, CIC_Decimation_Filter1/1(Input)
  In2/1 -> Scope1/2, CIC_Decimation_Filter2/1(Input)
  Real-Imag to Complex/1 -> Scope3/3, Product/1
  Data Type Conversion/1 -> Product/2
  Constant/1 -> Data Type Conversion/1
  Product/1 -> Data Type Conversion3/1
  CIC_Decimation_Filter2/1(Output) -> Scope1/1, Scope3/2, Real-Imag to Complex/2
  CIC_Decimation_Filter1/1(Output) -> Scope2/2, Scope3/1, Real-Imag to Complex/1
  Data Type Conversion3/1 -> TTD_Farrow1/1(In1), Scope/2
  TTD_Farrow1/1(Output) -> Output/1, Scope/1

== system beam_control_ic_rx/Digital_Compensation4 ==
  Input : Inport  Partition=on  PartitionDimension=1  PartitionWidth=1  PartitionOffset=0
  In2 : Inport  Port=2  Partition=on  PartitionDimension=1  PartitionWidth=1  PartitionOffset=0
  CIC_Decimation_Filter1 : Subsystem  Tag=FilterWizardSubSystem
      settings: ErrorFcn=dspFilterRealizedInBasicElemsAlgLoopErrFcnCallback
  CIC_Decimation_Filter2 : Subsystem  Tag=FilterWizardSubSystem
      settings: ErrorFcn=dspFilterRealizedInBasicElemsAlgLoopErrFcnCallback
  Constant : Constant
  Constant1 : Constant  Value=fraction_delay
  Data Type Conversion : DataTypeConversion  OutDataTypeStr=fixdt(1,16,0)  SaturateOnIntegerOverflow=off  RndMeth=Floor
  Data Type Conversion1 : DataTypeConversion  OutDataTypeStr=fixdt(1,16,6)  SaturateOnIntegerOverflow=off  RndMeth=Floor
  For Each : ForEach  DisableCoverage=on
  Product : Product
  Real-Imag to Complex : RealImagToComplex
  Scope : Scope  NumInputPorts=2
  Scope1 : Scope  NumInputPorts=2
  Variable Fractional Delay : dspsigops/Variable Fractional Delay  mode=OBSOLETE  modeActive=Linear  L=4  FarrowL=4  R=10  alpha=1  dmax=100  InputProcessing=Columns as channels (frame based)  ic=0  noDFT=off  fallbackFIR=Clip to the minimum value necessary for centered kernel  fallbackFarrow=Clip to the minimum value necessary for centered kernel  roundingMode=Zero  overflowMode=off
  Out1 : Outport  ConcatenationDimension=1
  wires:
  CIC_Decimation_Filter1/1(Output) -> Real-Imag to Complex/1
  CIC_Decimation_Filter2/1(Output) -> Real-Imag to Complex/2, Scope1/1
  Data Type Conversion1/1 -> Variable Fractional Delay/2
  Constant1/1 -> Data Type Conversion1/1
  Variable Fractional Delay/1 -> Scope/1, Out1/1
  Product/1 -> Scope/2, Variable Fractional Delay/1
  Constant/1 -> Data Type Conversion/1
  Data Type Conversion/1 -> Product/2
  Real-Imag to Complex/1 -> Product/1
  In2/1 -> CIC_Decimation_Filter2/1(Input), Scope1/2
  Input/1 -> CIC_Decimation_Filter1/1(Input)

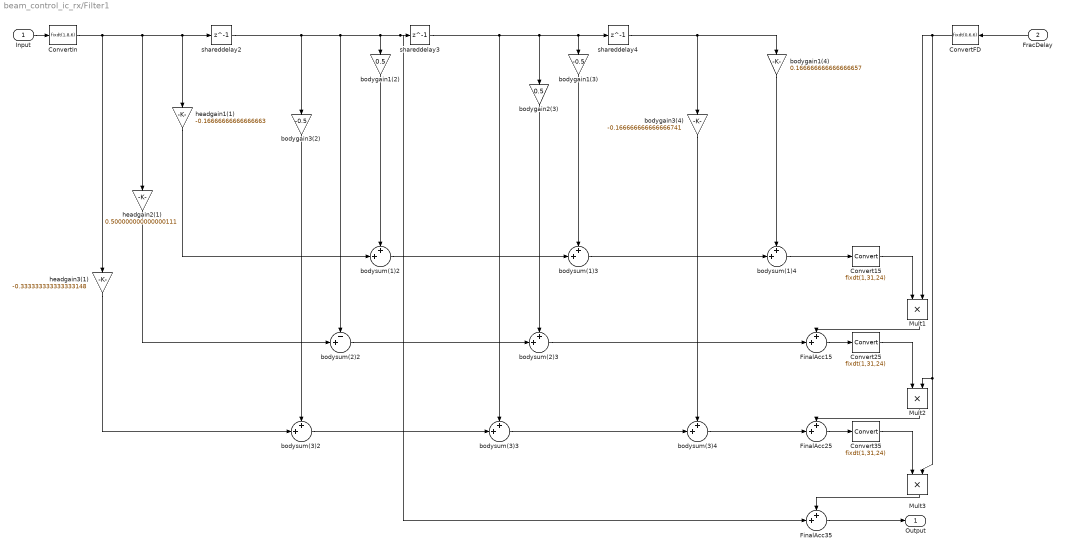
== system beam_control_ic_rx/Filter1 ==
  Input : Inport
  FracDelay : Inport  Port=2
  Convert15 : DataTypeConversion  OutDataTypeStr=fixdt(1,31,24)  RndMeth=Convergent  SaturateOnIntegerOverflow=off
  Convert25 : DataTypeConversion  OutDataTypeStr=fixdt(1,31,24)  RndMeth=Convergent  SaturateOnIntegerOverflow=off
  Convert35 : DataTypeConversion  OutDataTypeStr=fixdt(1,31,24)  RndMeth=Convergent  SaturateOnIntegerOverflow=off
  ConvertFD : DataTypeConversion  OutDataTypeStr=fixdt(0,6,6)  RndMeth=Nearest
  ConvertIn : DataTypeConversion  OutDataTypeStr=fixdt(1,8,6)  RndMeth=Nearest
  FinalAcc15 : Sum  Inputs=++|  AccumDataTypeStr=fixdt(1,38,30)  OutDataTypeStr=fixdt(1,38,30)  RndMeth=Convergent
  FinalAcc25 : Sum  Inputs=++|  AccumDataTypeStr=fixdt(1,38,30)  OutDataTypeStr=fixdt(1,38,30)  RndMeth=Convergent
  FinalAcc35 : Sum  Inputs=++|  AccumDataTypeStr=fixdt(1,38,30)  OutDataTypeStr=fixdt(1,38,30)  RndMeth=Convergent
  Mult1 : Product  OutDataTypeStr=fixdt(1,37,30)  RndMeth=Convergent
  Mult2 : Product  OutDataTypeStr=fixdt(1,37,30)  RndMeth=Convergent
  Mult3 : Product  OutDataTypeStr=fixdt(1,37,30)  RndMeth=Convergent
  bodygain1(2) : Gain  Gain=0.5  ParamDataTypeStr=fixdt(1,8,6)  OutDataTypeStr=fixdt(1,15,12)  RndMeth=Convergent
  bodygain1(3) : Gain  Gain=-0.5  ParamDataTypeStr=fixdt(1,8,6)  OutDataTypeStr=fixdt(1,15,12)  RndMeth=Convergent
  bodygain1(4) : Gain  Gain=0.166666666666666657  ParamDataTypeStr=fixdt(1,8,6)  OutDataTypeStr=fixdt(1,15,12)  RndMeth=Convergent
  bodygain2(3) : Gain  Gain=0.5  ParamDataTypeStr=fixdt(1,8,6)  OutDataTypeStr=fixdt(1,15,12)  RndMeth=Convergent
  bodygain3(2) : Gain  Gain=-0.5  ParamDataTypeStr=fixdt(1,8,6)  OutDataTypeStr=fixdt(1,15,12)  RndMeth=Convergent
  bodygain3(4) : Gain  Gain=-0.166666666666666741  ParamDataTypeStr=fixdt(1,8,6)  OutDataTypeStr=fixdt(1,15,12)  RndMeth=Convergent
  bodysum(1)2 : Sum  Inputs=++|  AccumDataTypeStr=fixdt(1,17,12)  OutDataTypeStr=fixdt(1,17,12)  RndMeth=Convergent
  bodysum(1)3 : Sum  Inputs=++|  AccumDataTypeStr=fixdt(1,17,12)  OutDataTypeStr=fixdt(1,17,12)  RndMeth=Convergent
  bodysum(1)4 : Sum  Inputs=++|  AccumDataTypeStr=fixdt(1,17,12)  OutDataTypeStr=fixdt(1,17,12)  RndMeth=Convergent
  bodysum(2)2 : Sum  Inputs=-+|  AccumDataTypeStr=fixdt(1,17,12)  OutDataTypeStr=fixdt(1,17,12)  RndMeth=Convergent
  bodysum(2)3 : Sum  Inputs=++|  AccumDataTypeStr=fixdt(1,17,12)  OutDataTypeStr=fixdt(1,17,12)  RndMeth=Convergent
  bodysum(3)2 : Sum  Inputs=++|  AccumDataTypeStr=fixdt(1,17,12)  OutDataTypeStr=fixdt(1,17,12)  RndMeth=Convergent
  bodysum(3)3 : Sum  Inputs=++|  AccumDataTypeStr=fixdt(1,17,12)  OutDataTypeStr=fixdt(1,17,12)  RndMeth=Convergent
  bodysum(3)4 : Sum  Inputs=++|  AccumDataTypeStr=fixdt(1,17,12)  OutDataTypeStr=fixdt(1,17,12)  RndMeth=Convergent
  headgain1(1) : Gain  Gain=-0.16666666666666663  ParamDataTypeStr=fixdt(1,8,6)  OutDataTypeStr=fixdt(1,15,12)  RndMeth=Convergent
  headgain2(1) : Gain  Gain=0.500000000000000111  ParamDataTypeStr=fixdt(1,8,6)  OutDataTypeStr=fixdt(1,15,12)  RndMeth=Convergent
  headgain3(1) : Gain  Gain=-0.333333333333333148  ParamDataTypeStr=fixdt(1,8,6)  OutDataTypeStr=fixdt(1,15,12)  RndMeth=Convergent
  shareddelay2 : Delay  DelayLength=1  InitialCondition=0  InputProcessing=Columns as channels (frame based)
  shareddelay3 : Delay  DelayLength=1  InitialCondition=0  InputProcessing=Columns as channels (frame based)
  shareddelay4 : Delay  DelayLength=1  InitialCondition=0  InputProcessing=Columns as channels (frame based)
  Output : Outport
  wires:
  headgain1(1)/1 -> bodysum(1)2/2
  headgain2(1)/1 -> bodysum(2)2/2
  headgain3(1)/1 -> bodysum(3)2/2
  Input/1 -> ConvertIn/1
  ConvertIn/1 -> headgain1(1)/1, shareddelay2/1, headgain2(1)/1, headgain3(1)/1
  bodygain1(2)/1 -> bodysum(1)2/1
  bodygain3(2)/1 -> bodysum(3)2/1
  bodysum(1)2/1 -> bodysum(1)3/2
  bodysum(2)2/1 -> bodysum(2)3/2
  bodysum(3)2/1 -> bodysum(3)3/2
  shareddelay2/1 -> FinalAcc35/2, shareddelay3/1, bodygain1(2)/1, bodysum(2)2/1, bodygain3(2)/1
  bodygain1(3)/1 -> bodysum(1)3/1
  bodygain2(3)/1 -> bodysum(2)3/1
  bodysum(1)3/1 -> bodysum(1)4/2
  bodysum(2)3/1 -> FinalAcc15/2
  bodysum(3)3/1 -> bodysum(3)4/2
  shareddelay3/1 -> bodygain1(3)/1, shareddelay4/1, bodygain2(3)/1, bodysum(3)3/1
  bodygain1(4)/1 -> bodysum(1)4/1
  bodygain3(4)/1 -> bodysum(3)4/1
  bodysum(1)4/1 -> Convert15/1
  bodysum(3)4/1 -> FinalAcc25/2
  shareddelay4/1 -> bodygain1(4)/1, bodygain3(4)/1
  FracDelay/1 -> ConvertFD/1
  ConvertFD/1 -> Mult2/2, Mult3/2, Mult1/2
  Convert15/1 -> Mult1/1
  Mult1/1 -> FinalAcc15/1
  FinalAcc15/1 -> Convert25/1
  Convert25/1 -> Mult2/1
  Mult2/1 -> FinalAcc25/1
  FinalAcc25/1 -> Convert35/1
  Convert35/1 -> Mult3/1
  Mult3/1 -> FinalAcc35/1
  FinalAcc35/1 -> Output/1

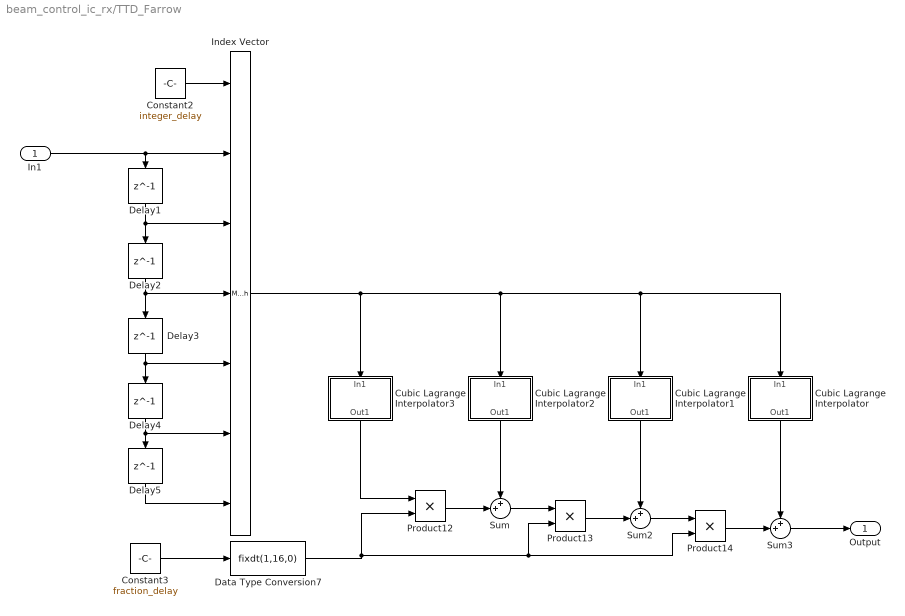
== system beam_control_ic_rx/TTD_Farrow ==
  In1 : Inport
  Constant2 : Constant  Value=integer_delay
  Constant3 : Constant  Value=fraction_delay
  Cubic Lagrange Interpolator : Subsystem
  Cubic Lagrange Interpolator1 : Subsystem
  Cubic Lagrange Interpolator2 : Subsystem
  Cubic Lagrange Interpolator3 : Subsystem
  Data Type Conversion7 : DataTypeConversion  OutDataTypeStr=fixdt(1,16,0)  SaturateOnIntegerOverflow=off  RndMeth=Floor
  Delay{1..5} (5 alike) : Delay  DelayLength=1
  Index Vector : MultiPortSwitch  DataPortOrder=Zero-based contiguous  Inputs=6  zeroidx=on  SaturateOnIntegerOverflow=off  InputSameDT=off
  Product12 : Product
  Product13 : Product
  Product14 : Product
  Sum : Sum  Inputs=++|
  Sum2 : Sum  Inputs=++|
  Sum3 : Sum  Inputs=++|
  Output : Outport
  wires:
  Data Type Conversion7/1 -> Product12/2, Product13/2, Product14/2
  Sum/1 -> Product13/1
  Product14/1 -> Sum3/2
  Cubic Lagrange Interpolator1/1(Out1) -> Sum2/1
  Product12/1 -> Sum/2
  Index Vector/1 -> Cubic Lagrange Interpolator3/1(In1), Cubic Lagrange Interpolator2/1(In1), Cubic Lagrange Interpolator1/1(In1), Cubic Lagrange Interpolator/1(In1)
  Constant2/1 -> Index Vector/1
  Delay5/1 -> Index Vector/7
  Cubic Lagrange Interpolator3/1(Out1) -> Product12/1
  Sum2/1 -> Product14/1
  Delay4/1 -> Index Vector/6, Delay5/1
  Delay3/1 -> Index Vector/5, Delay4/1
  Delay1/1 -> Index Vector/3, Delay2/1
  Product13/1 -> Sum2/2
  Delay2/1 -> Delay3/1, Index Vector/4
  In1/1 -> Index Vector/2, Delay1/1
  Sum3/1 -> Output/1
  Cubic Lagrange Interpolator/1(Out1) -> Sum3/1
  Cubic Lagrange Interpolator2/1(Out1) -> Sum/1
  Constant3/1 -> Data Type Conversion7/1

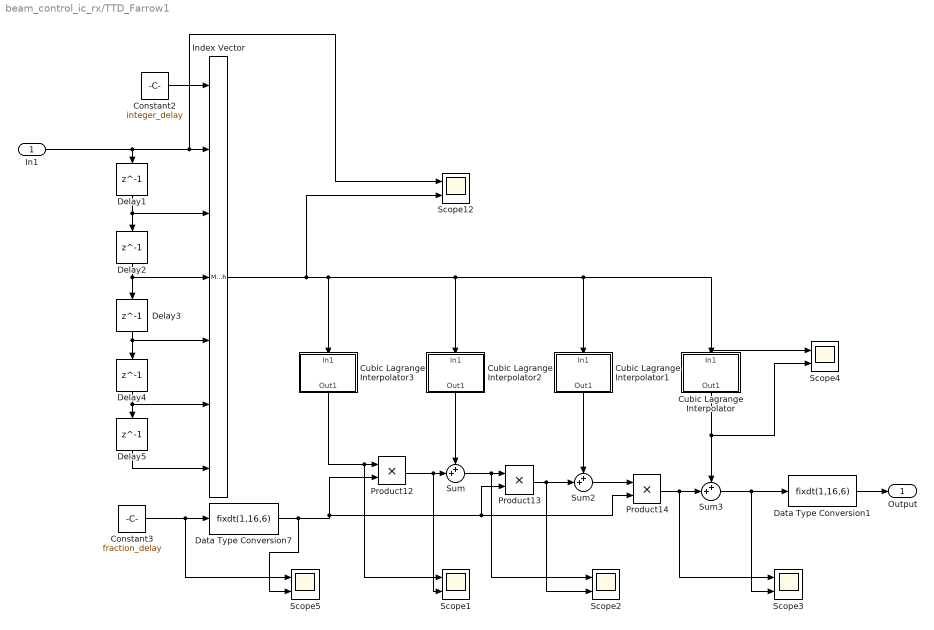
== system beam_control_ic_rx/TTD_Farrow1 ==
  In1 : Inport
  Constant2 : Constant  Value=integer_delay
  Constant3 : Constant  Value=fraction_delay
  Cubic Lagrange Interpolator : Subsystem
  Cubic Lagrange Interpolator1 : Subsystem
  Cubic Lagrange Interpolator2 : Subsystem
  Cubic Lagrange Interpolator3 : Subsystem
  Data Type Conversion1 : DataTypeConversion  OutDataTypeStr=fixdt(1,16,6)  SaturateOnIntegerOverflow=off  RndMeth=Floor
  Data Type Conversion7 : DataTypeConversion  OutDataTypeStr=fixdt(1,16,6)  SaturateOnIntegerOverflow=off  RndMeth=Floor
  Delay{1..5} (5 alike) : Delay  DelayLength=1
  Index Vector : MultiPortSwitch  DataPortOrder=Zero-based contiguous  Inputs=6  zeroidx=on  SaturateOnIntegerOverflow=off  InputSameDT=off
  Product12 : Product
  Product13 : Product
  Product14 : Product
  Scope{1..5,12} (6 alike) : Scope  NumInputPorts=2
  Sum : Sum  Inputs=++|
  Sum2 : Sum  Inputs=++|
  Sum3 : Sum  Inputs=++|
  Output : Outport
  wires:
  Data Type Conversion1/1 -> Output/1
  Data Type Conversion7/1 -> Product12/2, Product13/2, Product14/2, Scope5/2
  Sum/1 -> Product13/1, Scope2/1
  Product14/1 -> Sum3/2, Scope3/1
  Cubic Lagrange Interpolator1/1(Out1) -> Sum2/1
  Product12/1 -> Sum/2, Scope1/2
  Index Vector/1 -> Cubic Lagrange Interpolator3/1(In1), Cubic Lagrange Interpolator2/1(In1), Cubic Lagrange Interpolator1/1(In1), Cubic Lagrange Interpolator/1(In1), Scope4/1, Scope12/2
  Constant2/1 -> Index Vector/1
  Delay5/1 -> Index Vector/7
  Cubic Lagrange Interpolator3/1(Out1) -> Product12/1, Scope1/1
  Sum2/1 -> Product14/1
  Delay4/1 -> Index Vector/6, Delay5/1
  Delay3/1 -> Index Vector/5, Delay4/1
  Delay1/1 -> Index Vector/3, Delay2/1
  Product13/1 -> Sum2/2, Scope2/2
  Delay2/1 -> Delay3/1, Index Vector/4
  In1/1 -> Index Vector/2, Scope12/1, Delay1/1
  Sum3/1 -> Data Type Conversion1/1, Scope3/2
  Cubic Lagrange Interpolator/1(Out1) -> Sum3/1, Scope4/2
  Cubic Lagrange Interpolator2/1(Out1) -> Sum/1
  Constant3/1 -> Data Type Conversion7/1, Scope5/1

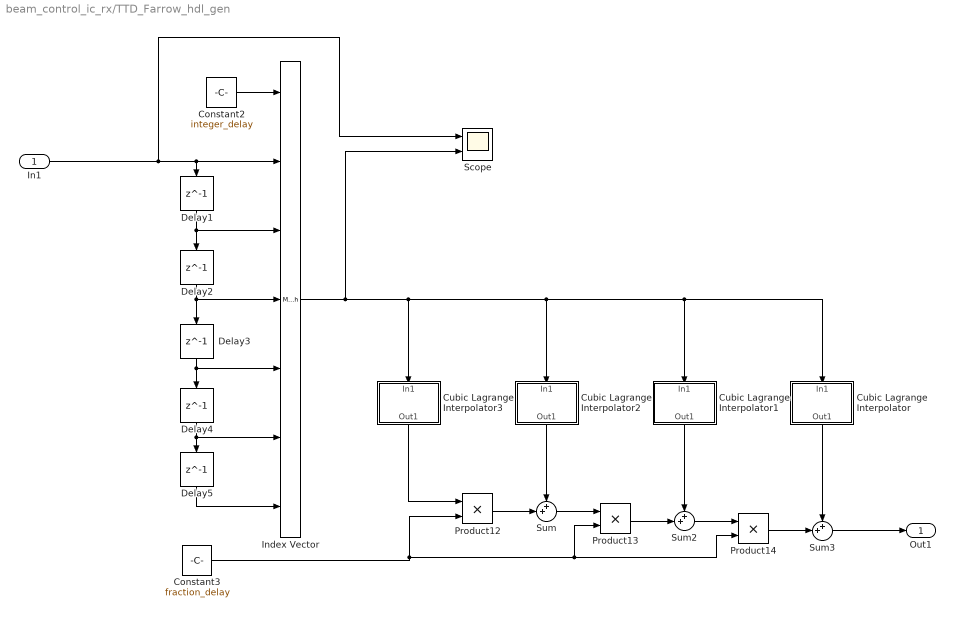
== system beam_control_ic_rx/TTD_Farrow_hdl_gen ==
  In1 : Inport
  Constant2 : Constant  Value=integer_delay  OutDataTypeStr=fixdt(1,16,0)
  Constant3 : Constant  Value=fraction_delay  OutDataTypeStr=fixdt(1,16,0)
  Cubic Lagrange Interpolator : Subsystem
  Cubic Lagrange Interpolator1 : Subsystem
  Cubic Lagrange Interpolator2 : Subsystem
  Cubic Lagrange Interpolator3 : Subsystem
  Delay{1..5} (5 alike) : Delay  DelayLength=1
  Index Vector : MultiPortSwitch  DataPortOrder=Zero-based contiguous  Inputs=6  zeroidx=on  SaturateOnIntegerOverflow=off  InputSameDT=off
  Product12 : Product
  Product13 : Product
  Product14 : Product
  Scope : Scope  NumInputPorts=2
  Sum : Sum  Inputs=++|
  Sum2 : Sum  Inputs=++|
  Sum3 : Sum  Inputs=++|
  Out1 : Outport
  wires:
  Cubic Lagrange Interpolator3/1(Out1) -> Product12/1
  In1/1 -> Scope/1, Delay1/1, Index Vector/2
  Constant3/1 -> Product14/2, Product13/2, Product12/2
  Index Vector/1 -> Scope/2, Cubic Lagrange Interpolator/1(In1), Cubic Lagrange Interpolator1/1(In1), Cubic Lagrange Interpolator2/1(In1), Cubic Lagrange Interpolator3/1(In1)
  Product14/1 -> Sum3/2
  Product13/1 -> Sum2/2
  Delay2/1 -> Index Vector/4, Delay3/1
  Cubic Lagrange Interpolator2/1(Out1) -> Sum/1
  Cubic Lagrange Interpolator1/1(Out1) -> Sum2/1
  Delay3/1 -> Delay4/1, Index Vector/5
  Sum/1 -> Product13/1
  Cubic Lagrange Interpolator/1(Out1) -> Sum3/1
  Product12/1 -> Sum/2
  Delay5/1 -> Index Vector/7
  Delay1/1 -> Delay2/1, Index Vector/3
  Sum2/1 -> Product14/1
  Sum3/1 -> Out1/1
  Delay4/1 -> Delay5/1, Index Vector/6
  Constant2/1 -> Index Vector/1

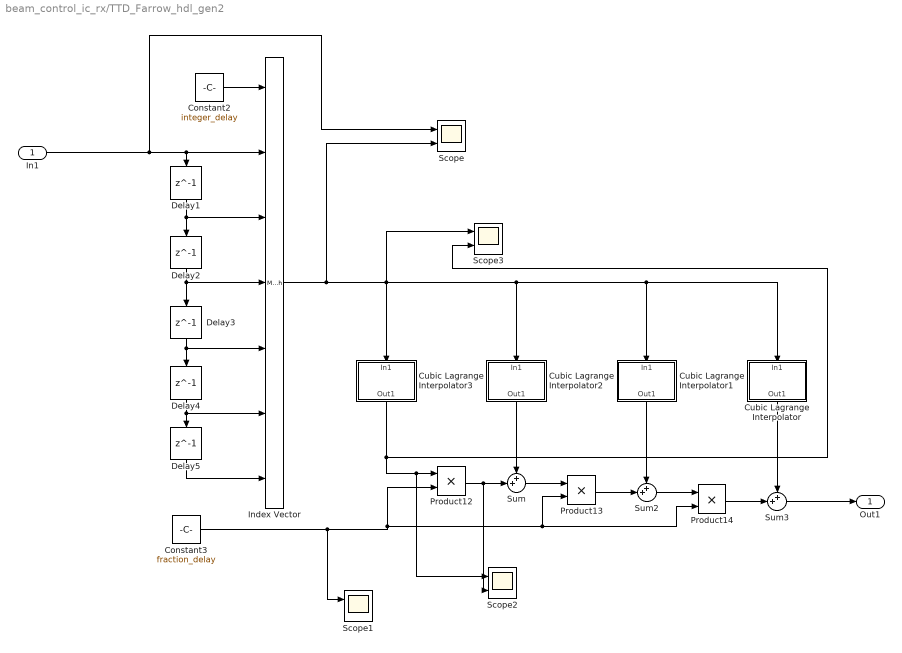
== system beam_control_ic_rx/TTD_Farrow_hdl_gen2 ==
  In1 : Inport
  Constant2 : Constant  Value=integer_delay  OutDataTypeStr=fixdt(1,16,0)
  Constant3 : Constant  Value=fraction_delay  OutMin=-10  OutMax=10  OutDataTypeStr=fixdt(1,16,10)
  Cubic Lagrange Interpolator : Subsystem
  Cubic Lagrange Interpolator1 : Subsystem
  Cubic Lagrange Interpolator2 : Subsystem
  Cubic Lagrange Interpolator3 : Subsystem
  Delay{1..5} (5 alike) : Delay  DelayLength=1
  Index Vector : MultiPortSwitch  DataPortOrder=Zero-based contiguous  Inputs=6  zeroidx=on  SaturateOnIntegerOverflow=off  InputSameDT=off
  Product12 : Product
  Product13 : Product
  Product14 : Product
  Scope{,1..3} (4 alike) : Scope  NumInputPorts=2
  Sum : Sum  Inputs=++|
  Sum2 : Sum  Inputs=++|
  Sum3 : Sum  Inputs=++|
  Out1 : Outport
  wires:
  Cubic Lagrange Interpolator3/1(Out1) -> Product12/1, Scope2/1, Scope3/2
  In1/1 -> Scope/1, Delay1/1, Index Vector/2
  Constant3/1 -> Product14/2, Product13/2, Product12/2, Scope1/1
  Index Vector/1 -> Scope/2, Cubic Lagrange Interpolator/1(In1), Cubic Lagrange Interpolator1/1(In1), Cubic Lagrange Interpolator2/1(In1), Scope3/1, Cubic Lagrange Interpolator3/1(In1)
  Product14/1 -> Sum3/2
  Product13/1 -> Sum2/2
  Delay2/1 -> Index Vector/4, Delay3/1
  Cubic Lagrange Interpolator2/1(Out1) -> Sum/1
  Cubic Lagrange Interpolator1/1(Out1) -> Sum2/1
  Delay3/1 -> Delay4/1, Index Vector/5
  Sum/1 -> Product13/1
  Cubic Lagrange Interpolator/1(Out1) -> Sum3/1
  Product12/1 -> Sum/2, Scope2/2
  Delay5/1 -> Index Vector/7
  Delay1/1 -> Delay2/1, Index Vector/3
  Sum2/1 -> Product14/1
  Sum3/1 -> Out1/1
  Delay4/1 -> Delay5/1, Index Vector/6
  Constant2/1 -> Index Vector/1
